simulink model "continuous_4_channel"  (R2020b)
settings: Solver=ode45  StartTime=0.0  StopTime=5  RelTol=1e-3
values from neighbouring files (symbols this model uses):
  Amp = 1    [hw1_main.m]
  Be = 0    [hw1_main.m]
  Bh = 1.5    [hw1_main.m]
  Bm = 0.8    [hw1_main.m]
  Bs = Bm*4    (= 3.2)    [hw1_main.m]
  Dh = 40    [hw1_main.m]
  Dm = 0    [hw1_main.m]
  Ds = 0    [hw1_main.m]
  Fc = 0.5    [hw1_main.m]
  Fip = 1    [hw1_main.m]
  Je = 0    [hw1_main.m]
  Jh = 0.5    [hw1_main.m]
  Ke = 200    [hw1_main.m]
  Kh = 1    [hw1_main.m]
  Km = 1    [hw1_main.m]
  Ks = Km*4    (= 4)    [hw1_main.m]
  Mm = 0.5    [hw1_main.m]
  Ms = 2    [hw1_main.m]
  Ph = 50    [hw1_main.m]
  xe = 0.5    [hw1_main.m]
settings Model: Creator=nicol  LastModifiedBy=nicol

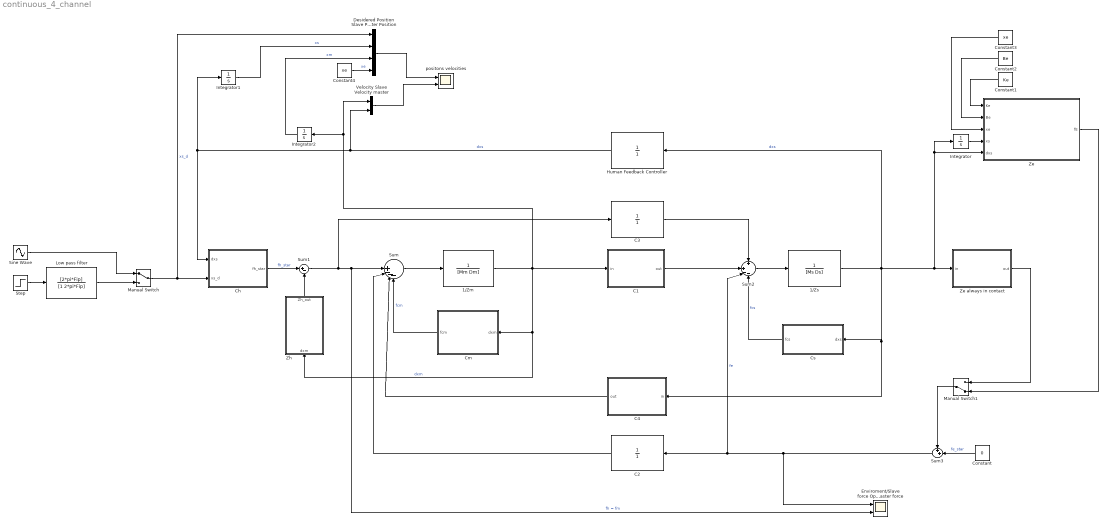
== system continuous_4_channel ==
  1/Zm : TransferFcn  Denominator=[Mm Dm]
  1/Zs : TransferFcn  Denominator=[Ms Ds]
  C1 : Subsystem
  C2 : TransferFcn  Denominator=[1]
  C3 : TransferFcn  Denominator=[1]
  C4 : Subsystem
  Ch : Subsystem
  Cm : Subsystem
  Constant : Constant  Value=0
  Constant1 : Constant  Value=Ke
  Constant2 : Constant  Value=Be
  Constant3 : Constant  Value=xe
  Constant4 : Constant  Value=xe
  Cs : Subsystem
  Desidered Position Slave Position Master Position : Mux
  Enviroment/Slave force Operator/Master force : Scope  NumInputPorts=2
  Human Feedback Controller : TransferFcn  Denominator=[1]
  Integrator : Integrator
  Integrator1 : Integrator
  Integrator2 : Integrator
  Low pass filter : TransferFcn  Numerator=[2*pi*Fip]  Denominator=[1 2*pi*Fip]
  Manual Switch : ManualSwitch
  Manual Switch1 : ManualSwitch  CurrentSetting=0
  Sine Wave : Sin  Amplitude=Amp  Frequency=2*pi*Fc  SampleTime=0
  Step : Step  After=Amp  SampleTime=0
  Sum : Sum  Inputs=|||+---
  Sum1 : Sum  Inputs=|+-
  Sum2 : Sum  Inputs=+|+--
  Sum3 : Sum  Inputs=++|
  Velocity Slave Velocity master : Mux  Inputs=2
  Ze : MATLAB Function  TreatAsAtomicUnit=on
  Ze always in contact : Subsystem
  Zh : Subsystem
  "positons velocities " : Scope  NumInputPorts=2
  wires:
  Sine Wave/1 -> Manual Switch/1
  Ch/1(fh_star) -> Sum1/1  "fh_star"
  Zh/1(Zh_out) -> Sum1/2
  1/Zm/1 -> Velocity Slave Velocity master/1, Integrator2/1, C1/1(in), Zh/1(dxm), Cm/1(dxm)  "dxm"
  Cm/1(fcm) -> Sum/4  "fcm"
  Sum1/1 -> C3/1, Enviroment/Slave force Operator/Master force/2, Sum/1  "fh = fm"
  C2/1 -> Sum/2
  C4/1(out) -> Sum/3
  C1/1(out) -> Sum2/2
  C3/1 -> Sum2/1
  Cs/1(fcs) -> Sum2/4  "fcs"
  1/Zs/1 -> C4/1(in), Cs/1(dxs), Human Feedback Controller/1, Ze always in contact/1(in), Ze/5(dxs), Integrator/1  "dxs"
  Sum2/1 -> 1/Zs/1
  Ze/1(fE) -> Manual Switch1/2
  Sum3/1 -> Enviroment/Slave force Operator/Master force/1, Sum2/3, C2/1  "fe"
  Human Feedback Controller/1 -> Velocity Slave Velocity master/2, Integrator1/1, Ch/1(dxs)  "dxs"
  Constant/1 -> Sum3/2  "fe_star"
  Constant1/1 -> Ze/1(Ke)
  Constant2/1 -> Ze/2(Be)
  Constant3/1 -> Ze/3(xe)
  Integrator/1 -> Ze/4(xs)
  Step/1 -> Low pass filter/1
  Manual Switch/1 -> Desidered Position Slave Position Master Position/1, Ch/2(xs_d)  "xs_d"
  Low pass filter/1 -> Manual Switch/2
  Manual Switch1/1 -> Sum3/1
  Ze always in contact/1(out) -> Manual Switch1/1
  Sum/1 -> 1/Zm/1
  Integrator1/1 -> Desidered Position Slave Position Master Position/2  "xs"
  Integrator2/1 -> Desidered Position Slave Position Master Position/3  "xm"
  Velocity Slave Velocity master/1 -> "positons velocities "/2
  Desidered Position Slave Position Master Position/1 -> "positons velocities "/1
  Constant4/1 -> Desidered Position Slave Position Master Position/4  "xe"

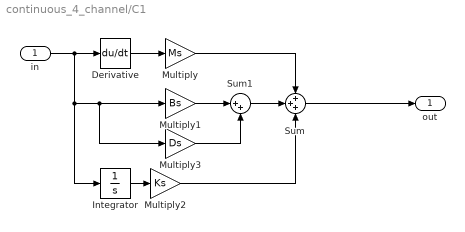
== system continuous_4_channel/C1 ==
  in : Inport
  Derivative : Derivative
  Integrator : Integrator
  Multiply : Gain  Gain=Ms
  Multiply1 : Gain  Gain=Bs
  Multiply2 : Gain  Gain=Ks
  Multiply3 : Gain  Gain=Ds
  Sum : Sum  Inputs=+++
  Sum1 : Sum  Inputs=|++
  out : Outport
  wires:
  in/1 -> Integrator/1, Multiply3/1, Multiply1/1, Derivative/1
  Derivative/1 -> Multiply/1
  Sum/1 -> out/1
  Integrator/1 -> Multiply2/1
  Multiply1/1 -> Sum1/1
  Multiply/1 -> Sum/1
  Multiply2/1 -> Sum/3
  Sum1/1 -> Sum/2
  Multiply3/1 -> Sum1/2

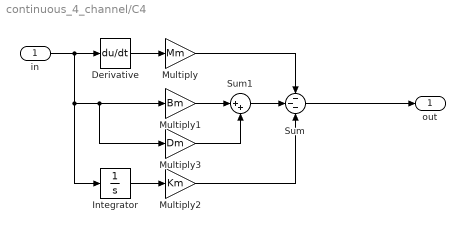
== system continuous_4_channel/C4 ==
  in : Inport
  Derivative : Derivative
  Integrator : Integrator
  Multiply : Gain  Gain=Mm
  Multiply1 : Gain  Gain=Bm
  Multiply2 : Gain  Gain=Km
  Multiply3 : Gain  Gain=Dm
  Sum : Sum  Inputs=---
  Sum1 : Sum  Inputs=|++
  out : Outport
  wires:
  in/1 -> Integrator/1, Multiply3/1, Multiply1/1, Derivative/1
  Derivative/1 -> Multiply/1
  Sum/1 -> out/1
  Integrator/1 -> Multiply2/1
  Multiply1/1 -> Sum1/1
  Multiply/1 -> Sum/1
  Multiply2/1 -> Sum/3
  Sum1/1 -> Sum/2
  Multiply3/1 -> Sum1/2

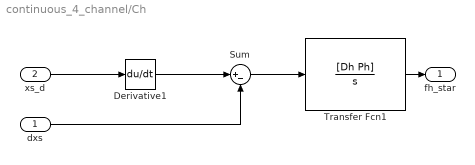
== system continuous_4_channel/Ch ==
  dxs : Inport
  xs_d : Inport  Port=2
  Derivative1 : Derivative
  Sum : Sum  Inputs=|+-
  Transfer Fcn1 : TransferFcn  Numerator=[Dh Ph]  Denominator=[1 0]
  fh_star : Outport
  wires:
  dxs/1 -> Sum/2
  Sum/1 -> Transfer Fcn1/1
  Transfer Fcn1/1 -> fh_star/1
  xs_d/1 -> Derivative1/1
  Derivative1/1 -> Sum/1

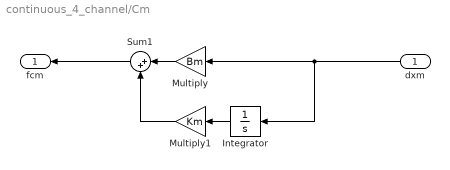
== system continuous_4_channel/Cm ==
  dxm : Inport
  Integrator : Integrator
  Multiply : Gain  Gain=Bm
  Multiply1 : Gain  Gain=Km
  Sum1 : Sum  Inputs=|++
  fcm : Outport
  wires:
  dxm/1 -> Integrator/1, Multiply/1
  Integrator/1 -> Multiply1/1
  Multiply1/1 -> Sum1/2
  Multiply/1 -> Sum1/1
  Sum1/1 -> fcm/1

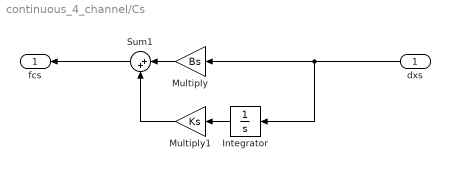
== system continuous_4_channel/Cs ==
  dxs : Inport
  Integrator : Integrator
  Multiply : Gain  Gain=Bs
  Multiply1 : Gain  Gain=Ks
  Sum1 : Sum  Inputs=|++
  fcs : Outport
  wires:
  dxs/1 -> Integrator/1, Multiply/1
  Integrator/1 -> Multiply1/1
  Multiply1/1 -> Sum1/2
  Multiply/1 -> Sum1/1
  Sum1/1 -> fcs/1

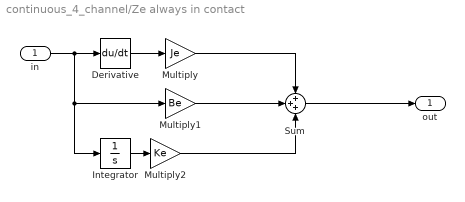
== system continuous_4_channel/Ze always in contact ==
  in : Inport
  Derivative : Derivative
  Integrator : Integrator
  Multiply : Gain  Gain=Je
  Multiply1 : Gain  Gain=Be
  Multiply2 : Gain  Gain=Ke
  Sum : Sum  Inputs=+++
  out : Outport
  wires:
  in/1 -> Integrator/1, Multiply1/1, Derivative/1
  Derivative/1 -> Multiply/1
  Sum/1 -> out/1
  Integrator/1 -> Multiply2/1
  Multiply1/1 -> Sum/2
  Multiply/1 -> Sum/1
  Multiply2/1 -> Sum/3

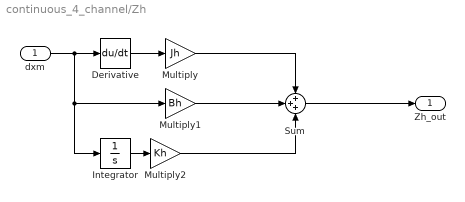
== system continuous_4_channel/Zh ==
  dxm : Inport
  Derivative : Derivative
  Integrator : Integrator
  Multiply : Gain  Gain=Jh
  Multiply1 : Gain  Gain=Bh
  Multiply2 : Gain  Gain=Kh
  Sum : Sum  Inputs=+++
  Zh_out : Outport
  wires:
  dxm/1 -> Integrator/1, Multiply1/1, Derivative/1
  Derivative/1 -> Multiply/1
  Sum/1 -> Zh_out/1
  Integrator/1 -> Multiply2/1
  Multiply1/1 -> Sum/2
  Multiply/1 -> Sum/1
  Multiply2/1 -> Sum/3

== matlab function continuous_4_channel/Ze ==
  data: Ke input; fE output; Be input; xe input; xs input; dxs input
function fE = environment(Ke, Be, xe, xs, dxs)
if(xs>xe)
    fE = Ke*(xs - xe) + Be*dxs;
else
    fE = 0;
end
